simulink model "MZexample"  (R2023a)
settings: Solver=FixedStepAuto  StartTime=0  StopTime=6.4583e-05  FixedStep=sample_time  RelTol=1e-3
model workspace: external: MAT-File D:\Roberto\Uni\DISPOSITIVI\modulator\matlab\values.mat (data not in the file)
values from neighbouring files (symbols this model uses):
  adj_frequency = frequency/prop_factor    (= 19354838.7097)    [initialValue.m]    (also in initial_value.m)
  delay_factor = 1/(2*pi*adj_frequency)    (= 8.22300539308e-09)    [initialValue.m]    (also in initial_value.m)
  gap = 6* um    (= 6e-06)    [MZS_ER_RF.m]    (also in MZS_ER_alpha.m; MZS_ER_kL.m; MZsimulation.m; initialValue.m)
  initial_buffer = 1024*100    (= 102400)    [initial_value.m]
  kL_factor_c = model_workspace.getVariable('kL_factor_c')    [LS_Base.m]    (also in LS_noise.m; MZS_ER_RF.m = kL_factor(k,2); MZS_ER_alpha.m = [pi/4, (pi/4)*1.10, (pi/4)*0.90, (pi/4)*1.5]; MZS_ER_kL.m = kL_factor_s/splitter_combiner_ratio)
  kL_factor_s = model_workspace.getVariable('kL_factor_s')    [LS_Base.m]    (also in LS_noise.m; MZS_ER_RF.m = kL_factor(k,1); MZS_ER_alpha.m = [pi/4, (pi/4)*1.10, (pi/4)*0.90, (pi/4)*1.5]; MZS_ER_kL.m = kL_factor(k))
  Length = 5* cm    (= 0.05)    [MZS_ER_RF.m]    (also in MZS_ER_alpha.m; MZS_ER_kL.m; MZsimulation.m; initialValue.m)
  loss_factor_1 = exp(-(loss_1/8.6860000037)*Length)    [initial_value.m]
  loss_factor_2 = exp(-(loss_2/8.6860000037)*Length)    [initial_value.m]
  pi_half_delay = time_delay(-pi/2, delay_factor)    [initialValue.m]    (also in initial_value.m)
  wavelength = 1550*nm    (= 1.55e-06)    [MZS_ER_RF.m]    (also in MZS_ER_alpha.m; MZS_ER_kL.m; MZsimulation.m; initial_value.m)
settings Model: SimulationMode=rapid-accelerator  Creator=rober  LastModifiedBy=rober
settings DebuggingCC: SignalInfNanChecking=warning  TimeAdjustmentMsg=warning  SingleTaskRateTransMsg=warning  UnconnectedInputMsg=warning  UnconnectedOutputMsg=warning  UnconnectedLineMsg=warning  UniqueDataStoreMsg=error
settings ModelReferenceCC: EnableRefExpFcnMdlSchedulingChecks=on
settings RTWCC: DLArmComputeVersion=19.05

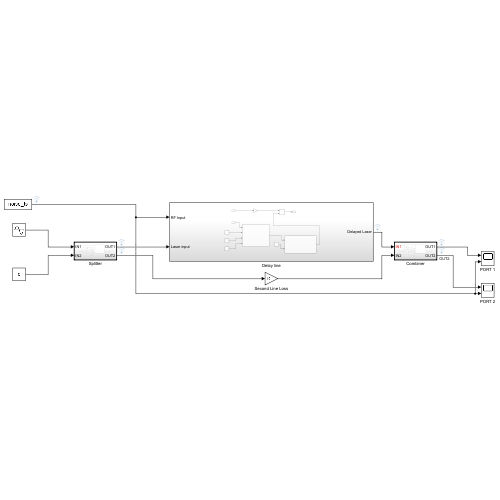
[thumbnail: Simulink's stored preview of the top-level diagram]
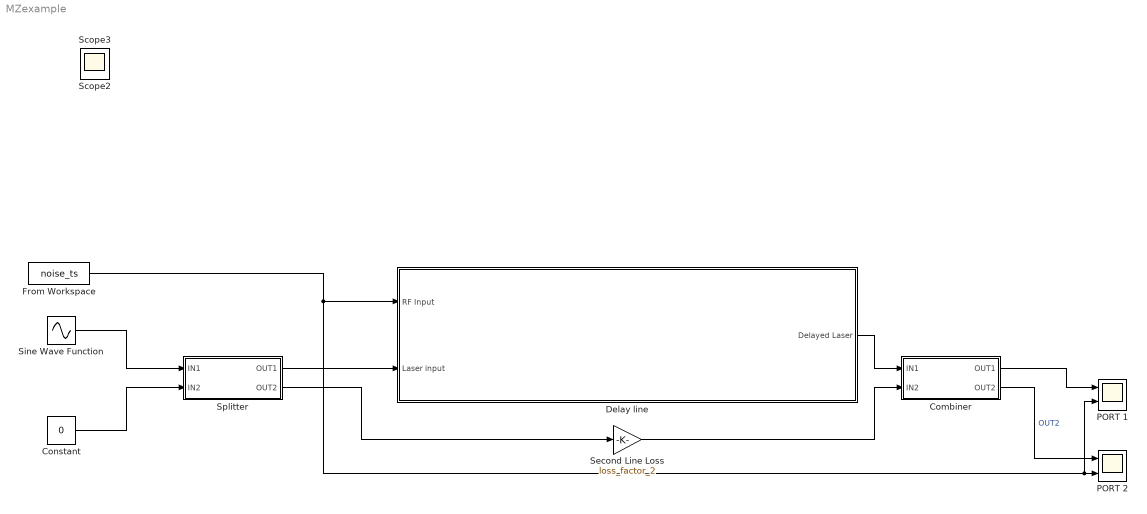
== system MZexample ==
  Combiner : Subsystem  TreatAsAtomicUnit=on
  Constant : Constant  Value=0
  Delay line : Subsystem
  From Workspace : FromWorkspace  VariableName=noise_ts
  PORT 1 : Scope  NumInputPorts=2
  PORT 2 : Scope  NumInputPorts=2
  Second Line Loss : Gain  Gain=loss_factor_2
  Sine Wave Function : Sin  Frequency=2*pi*adj_frequency  SampleTime=0
  Splitter : Subsystem  TreatAsAtomicUnit=on
  Scope2 : Scope
  Scope3 : Scope
  wires:
  From Workspace/1 -> PORT 1/2, PORT 2/2, Delay line/1("RF Input ")
  Delay line/1(Delayed Laser) -> Combiner/1(IN1)
  Splitter/1(OUT1) -> Delay line/2(Laser input)
  Sine Wave Function/1 -> Splitter/1(IN1)
  Constant/1 -> Splitter/2(IN2)
  Splitter/2(OUT2) -> Second Line Loss/1
  Combiner/2(OUT2) -> PORT 2/1  "OUT2"
  Combiner/1(OUT1) -> PORT 1/1
  Second Line Loss/1 -> Combiner/2(IN2)

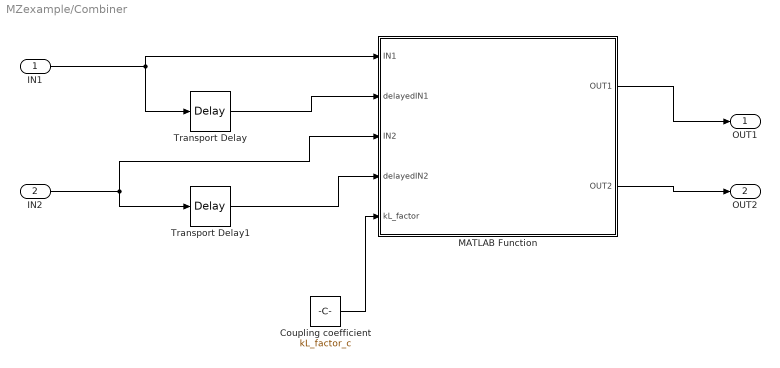
== system MZexample/Combiner ==
  IN1 : Inport
  IN2 : Inport  Port=2
  Coupling coefficient : Constant  Value=kL_factor_c
  MATLAB Function : MATLAB Function  TreatAsAtomicUnit=on
  Transport Delay : TransportDelay  DelayTime=pi_half_delay  BufferSize=initial_buffer  TransDelayFeedthrough=on
  Transport Delay1 : TransportDelay  DelayTime=pi_half_delay  BufferSize=initial_buffer  TransDelayFeedthrough=on
  OUT1 : Outport
  OUT2 : Outport  Port=2
  wires:
  IN1/1 -> Transport Delay/1, MATLAB Function/1(IN1)
  Transport Delay/1 -> MATLAB Function/2(delayedIN1)
  Transport Delay1/1 -> MATLAB Function/4(delayedIN2)
  IN2/1 -> Transport Delay1/1, MATLAB Function/3(IN2)
  MATLAB Function/1(OUT1) -> OUT1/1
  MATLAB Function/2(OUT2) -> OUT2/1
  Coupling coefficient/1 -> MATLAB Function/5(kL_factor)

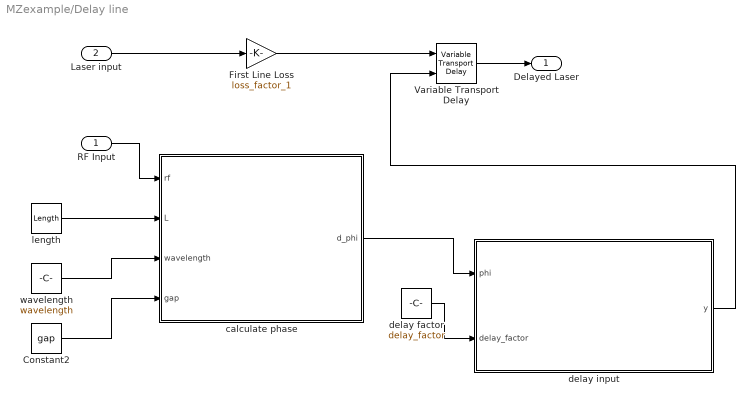
== system MZexample/Delay line ==
  "RF Input " : Inport
  Laser input : Inport  Port=2
  Constant2 : Constant  Value=gap
  First Line Loss : Gain  Gain=loss_factor_1
  Variable Transport Delay : VariableTransportDelay  MaximumDelay=maximun_time_delay  MaximumPoints=initial_buffer  ZeroDelay=on  TransDelayFeedthrough=on  PadeOrder=4
  calculate phase : MATLAB Function  TreatAsAtomicUnit=on
  delay factor : Constant  Value=delay_factor
  delay input : MATLAB Function  TreatAsAtomicUnit=on
  length : Constant  Value=Length
  wavelength : Constant  Value=wavelength
  Delayed Laser : Outport
  wires:
  "RF Input "/1 -> calculate phase/1(rf)
  calculate phase/1(d_phi) -> delay input/1(phi)
  delay input/1(y) -> Variable Transport Delay/2
  Variable Transport Delay/1 -> Delayed Laser/1
  wavelength/1 -> calculate phase/3(wavelength)
  length/1 -> calculate phase/2(L)
  Constant2/1 -> calculate phase/4(gap)
  delay factor/1 -> delay input/2(delay_factor)
  First Line Loss/1 -> Variable Transport Delay/1
  Laser input/1 -> First Line Loss/1

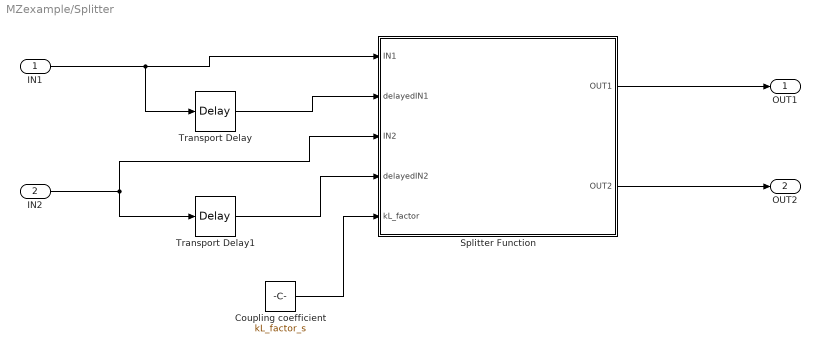
== system MZexample/Splitter ==
  IN1 : Inport
  IN2 : Inport  Port=2
  Coupling coefficient : Constant  Value=kL_factor_s
  Splitter Function : MATLAB Function  TreatAsAtomicUnit=on
  Transport Delay : TransportDelay  DelayTime=pi_half_delay  BufferSize=initial_buffer  TransDelayFeedthrough=on
  Transport Delay1 : TransportDelay  DelayTime=pi_half_delay  BufferSize=initial_buffer  TransDelayFeedthrough=on
  OUT1 : Outport
  OUT2 : Outport  Port=2
  wires:
  IN1/1 -> Transport Delay/1, Splitter Function/1(IN1)
  Transport Delay/1 -> Splitter Function/2(delayedIN1)
  Transport Delay1/1 -> Splitter Function/4(delayedIN2)
  IN2/1 -> Transport Delay1/1, Splitter Function/3(IN2)
  Splitter Function/1(OUT1) -> OUT1/1
  Splitter Function/2(OUT2) -> OUT2/1
  Coupling coefficient/1 -> Splitter Function/5(kL_factor)

== matlab function MZexample/Splitter/Splitter Function ==
  data: IN1 input; OUT1 output; OUT2 output; delayedIN1 input; IN2 input; delayedIN2 input; kL_factor input
function [OUT1, OUT2] = splitter(IN1, delayedIN1, IN2, delayedIN2, kL_factor)

OUT1 = cos(kL_factor)*IN1 + sin(kL_factor)*delayedIN2;
OUT2 = sin(kL_factor)*delayedIN1 + cos(kL_factor)*IN2;

== matlab function MZexample/Delay line/calculate phase ==
  data: d_phi output; rf input; L input; wavelength input; gap input
function d_phi = fcn( rf, L, wavelength, gap ) %in2 is left untouched 
    %%
    %Material : LiNbO3
    r33 = 30.8e-12;
    n0 = 2.2111;  
    confinment_factor = 0.32;
    %%
    n=n0-(n0^3)*r33*confinment_factor*rf/(2*gap);
    d_phi = ((2*pi)/wavelength)*(n0-n)*L;
end

== matlab function MZexample/Combiner/MATLAB Function ==
  data: IN1 input; OUT1 output; OUT2 output; delayedIN1 input; IN2 input; delayedIN2 input; kL_factor input
function [OUT1, OUT2] = splitter(IN1, delayedIN1, IN2, delayedIN2, kL_factor)

OUT1 = cos(kL_factor)*IN1 + sin(kL_factor)*delayedIN2;
OUT2 = sin(kL_factor)*delayedIN1 + cos(kL_factor)*IN2;

== matlab function MZexample/Delay line/delay input ==
  data: phi input; y output; delay_factor input
function y = fcn(phi, delay_factor)
y = time_delay(phi, delay_factor);
